simulink model "lab03z3_sch"  (R2021a)
settings: Solver=FixedStepAuto  StartTime=0.0  StopTime=10.0  FixedStep=0.01  RelTol=1e-3
values from neighbouring files (symbols this model uses):
  K = -place(A, B, s)    [lab03z3.m]
settings Model: Creator=user  LastModifiedBy=AgraWoodAdmin
settings SolverCC: AlgebraicLoopSolver=TrustRegion
settings DataIOCC: ReturnWorkspaceOutputs=off
settings DebuggingCC: SFMachineParentedDataDiag=warning  ArithmeticOperatorsInVariantConditions=warning
settings SFSimCC: SimUseLocalCustomCode=off  CustomCodeUndefinedFunction=UseInterfaceOnly
settings RTWCC: RTWUseLocalCustomCode=off

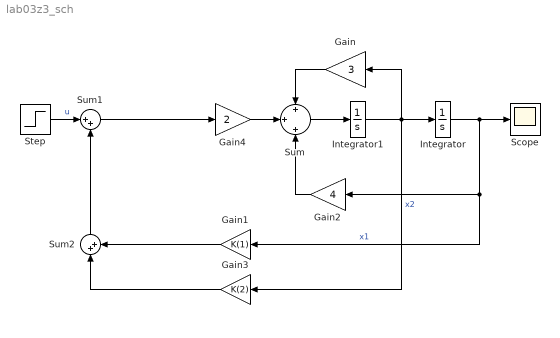
== system lab03z3_sch ==
  Gain : Gain  Gain=3
  Gain1 : Gain  Gain=K(1)
  Gain2 : Gain  Gain=4
  Gain3 : Gain  Gain=K(2)
  Gain4 : Gain  Gain=2
  Integrator : Integrator
  Integrator1 : Integrator
  Scope : Scope
  Step : Step  Time=0  After=10  SampleTime=0
  Sum : Sum  Inputs=+|+|+
  Sum1 : Sum  Inputs=|++
  Sum2 : Sum  Inputs=|++
  wires:
  Sum/1 -> Integrator1/1
  Gain/1 -> Sum/1
  Integrator1/1 -> Gain3/1, Integrator/1, Gain/1  "x2"
  Integrator/1 -> Scope/1, Gain1/1, Gain2/1  "x1"
  Gain2/1 -> Sum/3
  Gain4/1 -> Sum/2
  Sum1/1 -> Gain4/1
  Step/1 -> Sum1/1  "u"
  Gain1/1 -> Sum2/2
  Gain3/1 -> Sum2/1
  Sum2/1 -> Sum1/2
  ? -> ?  "x2"
